simulink model "se_pll_reduced_order_model"  (R2026a)
settings: Solver=ode45  StopTime=2.0  MaxStep=1e-3
undefined symbols (not defined in the file or in its folder): activePowerBias, activePowerScales, modalFrequency, zeta
settings Model: Creator=yao  LastModifiedBy=yao

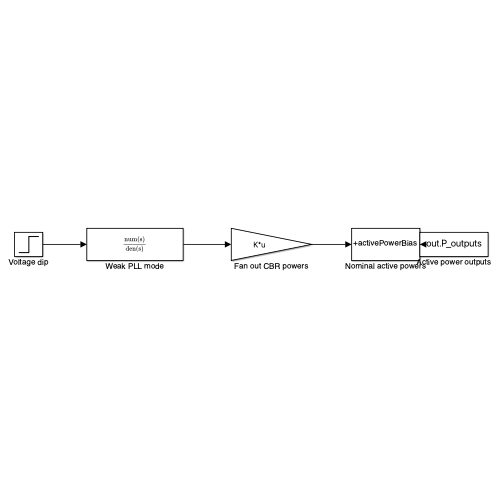
[thumbnail: Simulink's stored preview of the top-level diagram]
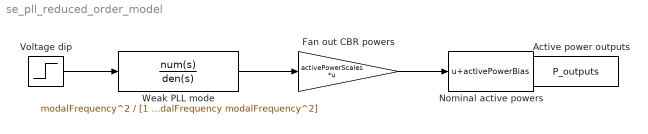
== system se_pll_reduced_order_model ==
  Active power outputs : ToWorkspace  VariableName=P_outputs  SaveFormat=Timeseries  SampleTime=-1
  Fan out CBR powers : Gain  Gain=activePowerScales  Multiplication=Matrix(K*u)
  Nominal active powers : Bias  Bias=activePowerBias  SaturateOnIntegerOverflow=off
  Voltage dip : Step  Time=0.10  FinalValue=disturbanceAmplitude  SampleTime=0
  Weak PLL mode : TransferFcn  Numerator=modalFrequency^2  Denominator=[1 2*zeta*modalFrequency modalFrequency^2]
  wires:
  Voltage dip/1 -> Weak PLL mode/1
  Weak PLL mode/1 -> Fan out CBR powers/1
  Fan out CBR powers/1 -> Nominal active powers/1
  Nominal active powers/1 -> Active power outputs/1
